simulink model "ExitEntrySend_2018a"  (R2018a)
settings: Solver=VariableStepAuto  StartTime=0.0  StopTime=10.0  RelTol=1e-3
settings Model: Creator=apple  LastModifiedBy=apple
settings DataIOCC: ReturnWorkspaceOutputs=on
settings SFSimCC: SimUseLocalCustomCode=on
settings RTWCC: RTWUseLocalCustomCode=on

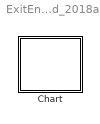
== system ExitEntrySend_2018a ==
  Chart : Stateflow chart  TreatAsAtomicUnit=on

== stateflow chart ExitEntrySend_2018a/Chart ==
  state B
    en:fprintf("Entry B");send(F);
    du:fprintf("During B");
    ex:fprintf("Exit B");
    state B1
      en:fprintf("Entry B1");
      du:fprintf("During B1");
      ex:fprintf("Exit B1");
    state B2
      en:fprintf("Entry B2");
      du:fprintf("During B2");
      ex:fprintf("Exit B2");
    (default) -> B1
  state A
    en:fprintf("Entry A");
    du:fprintf("During A");
    ex:fprintf("Exit A");
    state A1
      en:fprintf("Entry A1");
      du:fprintf("During A1");
      ex:fprintf("Exit A1");send(F);
    (default) -> A1
  (default) -> A
  A1 -> B2 : E/{fprintf("Transition Action1");}
  B2 -> A : F/{fprintf("Transition Action2");}
  events: E local FUNCTION_CALL_EVENT; F local FUNCTION_CALL_EVENT
